simulink model "Tx_Rx_BPSK_delta_simulatie"  (Simulink 7.4)
settings: Solver=ode45  StartTime=0.0  StopTime=inf  RelTol=1e-3
undefined symbols (not defined in the file): get
libraries: dspbuff3 x16, dsparch4 x6, simulink x6, commutil2 x4, dspsrcs4 x3, commfilt2 x3, dspsnks4 x2, commchan3 x1, commsink2 x1, dspmlti4 x1, commtimrec2 x1
settings Model: Creator=wnieves  LastModifiedBy=Bscheers
settings OptimizationCC: InitFltsAndDblsToZero=on

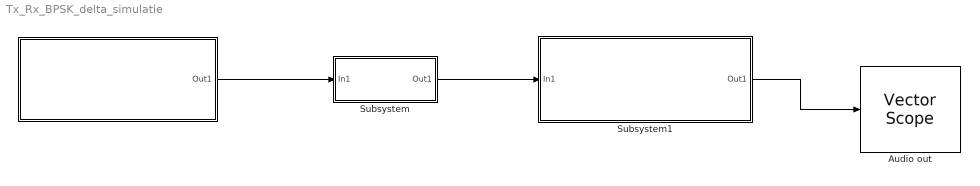
== system Tx_Rx_BPSK_delta_simulatie ==
  " " : Subsystem  Description=Transmitter
      mask Display: color('red');fprintf('Transmitter')
  Audio out : dspsnks4/Vector Scope  DialogController=dspdialog.VectorScope  DialogControllerArgs=DataTag7  ScopeProperties=on  Domain=Time  HorizSpan=1  DisplayProperties=off  AxisGrid=on  Memory=off  FrameNumber=on  AxisLegend=off  AxisZoom=off  OpenScopeAtSimStart=on  OpenScopeImmediately=off  FigPos=get(0,'defaultfigureposition')  AxisProperties=off  XUnits=Hertz  XRange=[0...Fs/2]  InheritXIncr=on  XIncr=1  XLabel=Time  XLimit=Auto  XMin=0  XMax=1  XStart=0  YUnits=dB  YLabel=Amplitude  LineProperties=off  XAxisParamsVer=6.9
      settings: YMin=-1  YMax=1
  Subsystem : Subsystem
      mask Display: fprintf('Channel')
  Subsystem1 : Subsystem
      mask Display: fprintf('Receiver')
  wires:
  " "/1(Out1) -> Subsystem/1(In1)
  Subsystem/1(Out1) -> Subsystem1/1(In1)
  Subsystem1/1(Out1) -> Audio out/1

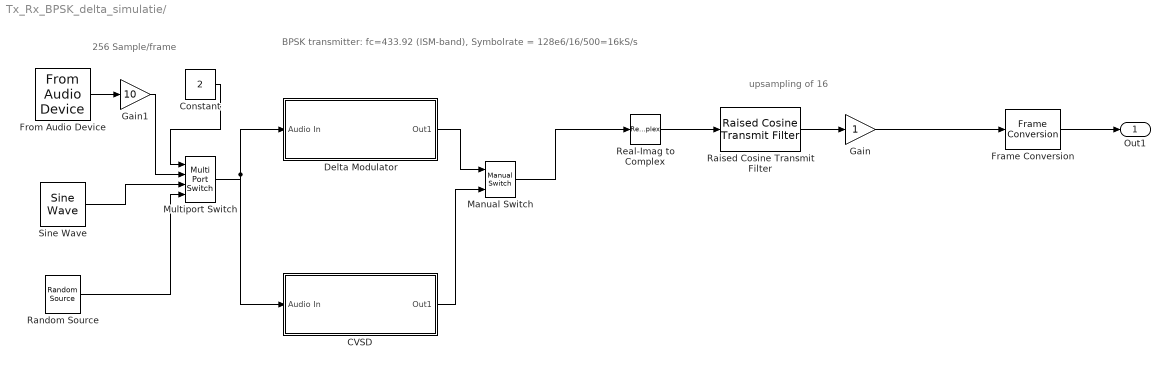
== system Tx_Rx_BPSK_delta_simulatie/  ==
  note: BPSK transmitter: fc=433.92 (ISM-band), Symbolrate = 128e6/16/500=16kS/s
  note: 256 Sample/frame
  note: upsampling of 16
  CVSD : Subsystem
  Constant : Constant  Value=2  OutDataType=fixdt(1, 16)  OutScaling=2^0
  Delta Modulator : Subsystem
  Frame Conversion : FrameConversion
  From Audio Device : dspsrcs4/From Audio Device  DialogController=dspDDGCreate  DialogControllerArgs=DataTag4  deviceName=Default  numChannels=1  sampleRate=16000  deviceDatatype=Determine from output data type  autoBufferSize=on  bufferSize=4096  queueDuration=1.0  frameSize=256  outputDatatype=single
  Gain : Gain  ParameterDataType=sfix(16)  ParameterScaling=2^0  OutDataType=sfix(16)  OutScaling=2^0
  Gain1 : Gain  Gain=10  ParameterDataType=fixdt(1, 16)  ParameterScaling=2^0  OutDataType=fixdt(1, 16)  OutScaling=2^0
  Manual Switch : simulink/Signal Routing/Manual Switch  SystemSampleTime=-1  sw=1  action=0  varsize=off
  Multiport Switch : MultiPortSwitch  OutDataType=fixdt(1, 16)  OutScaling=2^0
  Raised Cosine Transmit Filter : commfilt2/Raised Cosine Transmit Filter  DialogController=dspDDGCreate  DialogControllerArgs=DataTag5  SystemSampleTime=-1  filtType=Square root  D=8  R=0.35  sampMode=Mute  saveAsFlag=0  framing=Maintain input frame rate  N=16  checkGain=Normalized  filterGain=1  checkCoeff=off  variableName=rcTxFilt  launchFVT=off  roundingMode=Floor  overflowMode=off
  Random Source : dspsrcs4/Random Source  SrcType=Uniform  NormMethod=Ziggurat  CltLength=12  MinVal=-1  MaxVal=1  MeanVal=0  VarVal=1  RepMode=Not repeatable  rawSeed=1  IsInherit=off  SampMode=Discrete  SampTime=1/16000  SampFrame=256  DataType=Double  OutComplex=Real
  Real-Imag to Complex : RealImagToComplex  Input=Real
  Sine Wave : dspsrcs4/Sine Wave  Amplitude=1  Frequency=800  Phase=0  SampleMode=Discrete  OutComplex=Real  CompMethod=Trigonometric fcn  TableSize=Speed  SampleTime=1/16000  SamplesPerFrame=256  dataType=double  wordLen=16  udDataType=sfix(16)  fracBitsMode=Best precision  numFracBits=15  ResetState=Restart at time zero
  Out1 : Outport
  wires:
  Real-Imag to Complex/1 -> Raised Cosine Transmit Filter/1
  From Audio Device/1 -> Gain1/1
  Gain/1 -> Frame Conversion/1
  Raised Cosine Transmit Filter/1 -> Gain/1
  Delta Modulator/1(Out1) -> Manual Switch/1
  CVSD/1(Out1) -> Manual Switch/2
  Manual Switch/1 -> Real-Imag to Complex/1
  Frame Conversion/1 -> Out1/1
  Multiport Switch/1 -> Delta Modulator/1(Audio In), CVSD/1(Audio In)
  Gain1/1 -> Multiport Switch/2
  Sine Wave/1 -> Multiport Switch/3
  Random Source/1 -> Multiport Switch/4
  Constant/1 -> Multiport Switch/1

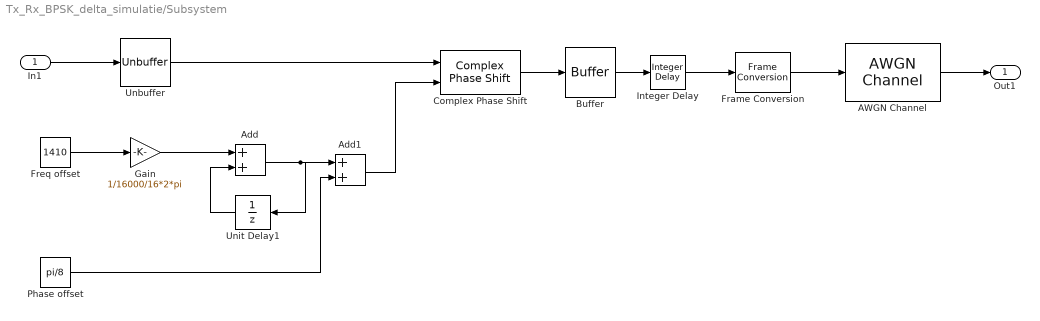
== system Tx_Rx_BPSK_delta_simulatie/Subsystem ==
  In1 : Inport  OutDataType=fixdt(1, 16)  OutScaling=2^0
  AWGN Channel : commchan3/AWGN Channel  SystemSampleTime=-1  seed=67  noiseMode="Signal to noise ratio  (SNR)"  EbNodB=20  EsNodB=10  SNRdB=20  bitsPerSym=1  Ps=1  Tsym=1  variance=1
  Add : Sum  OutDataType=fixdt(1, 16)  OutScaling=2^-10
  Add1 : Sum  OutDataType=fixdt(1, 16)  OutScaling=2^-10
  Buffer : dspbuff3/Buffer  N=4096  V=0  ic=0
  Complex Phase Shift : commutil2/Complex Phase Shift  SystemSampleTime=-1
  Frame Conversion : FrameConversion
  Freq offset : Constant  Value=1410  OutDataType=fixdt(1, 16)  OutScaling=2^0
      settings: SamplingMode=Frame based
  Gain : Gain  Gain=1/16000/16*2*pi  ParameterDataType=fixdt(1, 16)  ParameterScaling=2^0  OutDataType=fixdt(1, 16)  OutScaling=2^0
  Integer Delay : simulink/Discrete/Integer Delay  vinit=0.0  samptime=-1  NumDelays=4
  Phase offset : Constant  Value=pi/8  OutDataType=fixdt(1, 16)  OutScaling=2^0
      settings: SamplingMode=Frame based
  Unbuffer : dspbuff3/Unbuffer  ic=0
  Unit Delay1 : UnitDelay  SampleTime=-1
  Out1 : Outport  OutDataType=fixdt(1, 16)  OutScaling=2^0
  wires:
  Integer Delay/1 -> Frame Conversion/1
  Frame Conversion/1 -> AWGN Channel/1
  Complex Phase Shift/1 -> Buffer/1
  In1/1 -> Unbuffer/1
  Freq offset/1 -> Gain/1
  Gain/1 -> Add/1
  Add/1 -> Unit Delay1/1, Add1/1
  Unit Delay1/1 -> Add/2
  Phase offset/1 -> Add1/2
  Unbuffer/1 -> Complex Phase Shift/1
  Add1/1 -> Complex Phase Shift/2
  Buffer/1 -> Integer Delay/1
  AWGN Channel/1 -> Out1/1

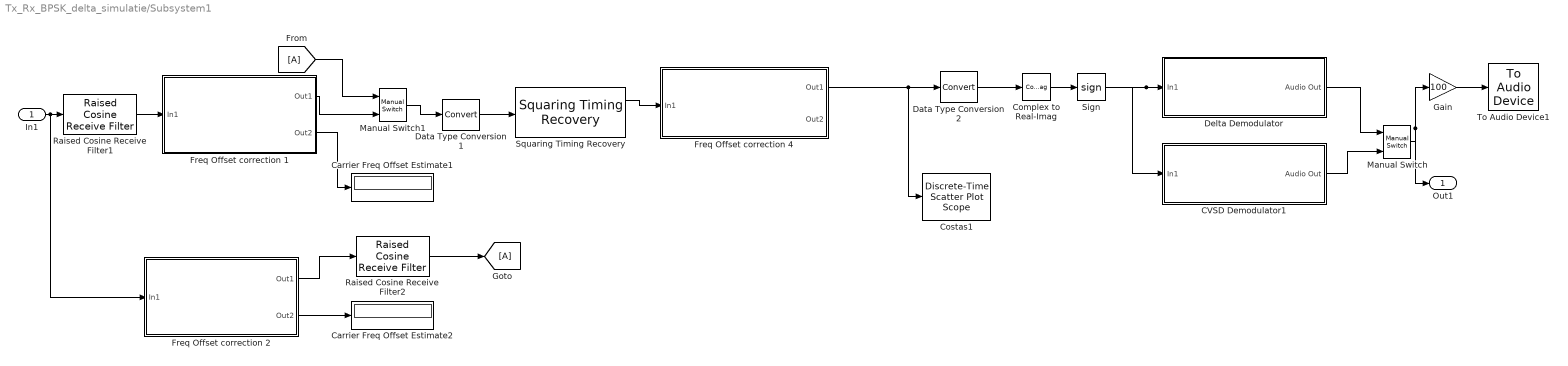
== system Tx_Rx_BPSK_delta_simulatie/Subsystem1 ==
  In1 : Inport  OutDataType=fixdt(1, 16)  OutScaling=2^0
  CVSD Demodulator1 : Subsystem
  Carrier Freq Offset Estimate1 : Display
  Carrier Freq Offset Estimate2 : Display
  Complex to Real-Imag : ComplexToRealImag  Output=Real
  Costas1 : commsink2/Discrete-Time Scatter Plot Scope  Tag=ScatterPlot  SystemSampleTime=-1  sampPerSymb=1  offsetEye=0  numTraces=40  numNewFrames=10  LineMarkers=.  LineColors=b  fading=on  render=on  AxisGrid=on  xMin=-1.60978085285153  xMax=1.62663894428818  yMin=-1.63581285423745  yMax=1.60060694290226  inphaseLabel=In-phase Amplitude  quadratureLabel=Quadrature Amplitude  openScopeAtSimStart=on  FrameNumber=off  FigPos=get(0,'defaultfigureposition');  figTitle=Scatter Plot  numLinesMax=8  block_type_=scatter
  Data Type Conversion1 : DataTypeConversion  OutDataType=fixdt(1, 16)  OutScaling=2^0
  Data Type Conversion2 : DataTypeConversion  OutDataType=fixdt(1, 16)  OutScaling=2^0
  Delta Demodulator : Subsystem
  Freq Offset correction 1 : Subsystem
      mask Display: fprintf('Delay and Multiply');
  Freq Offset correction 2 : Subsystem
      mask Display: fprintf('Coarse Freq Offset Estimater \n Delay-and-Multiply')
  Freq Offset correction 4 : Subsystem
      mask Display: fprintf('Costas Loop');
  Gain : Gain  Gain=100  ParameterDataType=fixdt(1, 16)  ParameterScaling=2^0  OutDataType=fixdt(1, 16)  OutScaling=2^0
  Manual Switch : simulink/Signal Routing/Manual Switch  SystemSampleTime=-1  sw=1  action=0  varsize=off
  Manual Switch1 : simulink/Signal Routing/Manual Switch  SystemSampleTime=-1  sw=0  action=0  varsize=off
  Raised Cosine Receive Filter1 : commfilt2/Raised Cosine Receive Filter  DialogController=dspDDGCreate  DialogControllerArgs=DataTag11  SystemSampleTime=-1  filtType=Square root  N=16  D=8  R=0.35  sampMode=Mute  saveAsFlag=0  framing=Maintain input frame rate  rateMode=None  downFactor=8  downOffset=0  checkGain=Normalized  filterGain=1  checkCoeff=off  variableName=rcRxFilt1  launchFVT=off  roundingMode=Floor  overflowMode=off
  Raised Cosine Receive Filter2 : commfilt2/Raised Cosine Receive Filter  DialogController=dspDDGCreate  DialogControllerArgs=DataTag12  SystemSampleTime=-1  filtType=Square root  N=16  D=8  R=0.35  sampMode=Mute  saveAsFlag=0  framing=Maintain input frame rate  rateMode=None  downFactor=8  downOffset=0  checkGain=Normalized  filterGain=1  checkCoeff=off  variableName=rcRxFilt2  launchFVT=off  roundingMode=Floor  overflowMode=off
  Sign : Signum
  Squaring Timing Recovery : commtimrec2/Squaring Timing Recovery  SystemSampleTime=-1  numSymb=256  sampPerSymb=16
  To Audio Device1 : dspsnks4/To Audio Device  DialogController=dspDDGCreate  DialogControllerArgs=DataTag13  deviceName=Default  inheritSampleRate=off  sampleRate=16000  deviceDatatype=Determine from input data type  autoBufferSize=on  bufferSize=4096  queueDuration=1.0
  Out1 : Outport  OutDataType=fixdt(1, 16)  OutScaling=2^0
  wires:
  Gain/1 -> To Audio Device1/1
  Delta Demodulator/1(Audio Out) -> Manual Switch/1
  Complex to Real-Imag/1 -> Sign/1
  Sign/1 -> Delta Demodulator/1(In1), CVSD Demodulator1/1(In1)
  Manual Switch/1 -> Gain/1, Out1/1
  CVSD Demodulator1/1(Audio Out) -> Manual Switch/2
  In1/1 -> Raised Cosine Receive Filter1/1, Freq Offset correction 2/1(In1)
  Freq Offset correction 1/2(Out2) -> Carrier Freq Offset Estimate1/1
  Freq Offset correction 2/2(Out2) -> Carrier Freq Offset Estimate2/1
  Raised Cosine Receive Filter1/1 -> Freq Offset correction 1/1(In1)
  Data Type Conversion1/1 -> Squaring Timing Recovery/1
  Freq Offset correction 2/1(Out1) -> Raised Cosine Receive Filter2/1
  Raised Cosine Receive Filter2/1 -> [A]
  Freq Offset correction 1/1(Out1) -> Manual Switch1/2
  Manual Switch1/1 -> Data Type Conversion1/1
  [A] -> Manual Switch1/1
  Freq Offset correction 4/1(Out1) -> Costas1/1, Data Type Conversion2/1
  Data Type Conversion2/1 -> Complex to Real-Imag/1
  Squaring Timing Recovery/1 -> Freq Offset correction 4/1(In1)

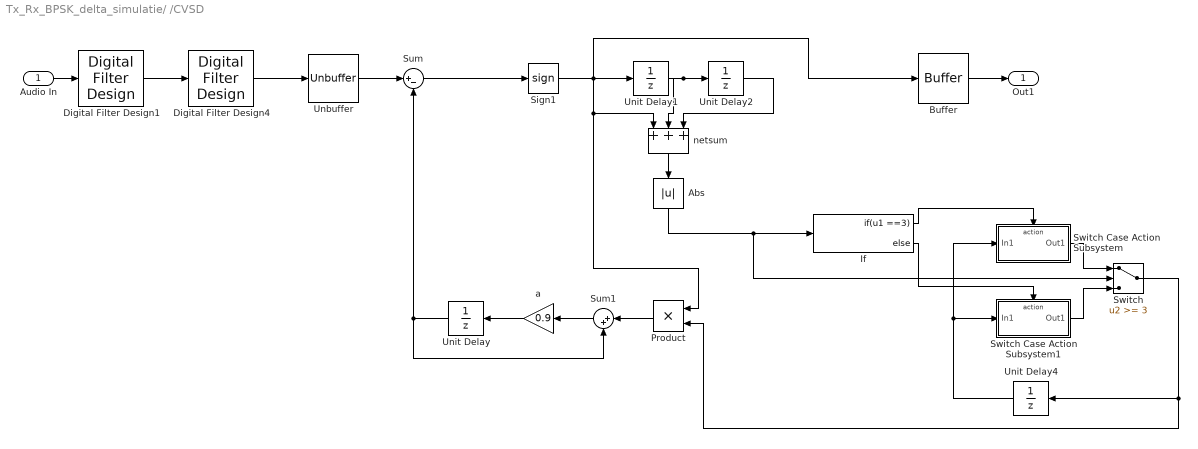
== system Tx_Rx_BPSK_delta_simulatie/ /CVSD ==
  Audio In : Inport
  Abs : Abs  OutDataType=fixdt(1, 16)  OutScaling=2^0
  Buffer : dspbuff3/Buffer  N=256  V=0  ic=0
  Digital Filter Design1 : dsparch4/Digital Filter Design  SystemSampleTime=-1  mwdsp_browser_bugfix_var=off
  Digital Filter Design4 : dsparch4/Digital Filter Design  SystemSampleTime=-1  mwdsp_browser_bugfix_var=off
  If : If  IfExpression=u1 ==3
  Product : Product  OutDataType=fixdt(1, 16)  OutScaling=2^0  RndMeth=Zero
  Sign1 : Signum
  Sum : Sum  Inputs=|+-  OutDataType=sfix(16)  OutScaling=2^0
  Sum1 : Sum  Inputs=|++  OutDataType=sfix(16)  OutScaling=2^0
  Switch : Switch  Threshold=3  OutDataType=fixdt(1, 16)  OutScaling=2^0
  Switch Case Action Subsystem : Subsystem  TreatAsAtomicUnit=on
  Switch Case Action Subsystem1 : Subsystem  TreatAsAtomicUnit=on
  Unbuffer : dspbuff3/Unbuffer  ic=0
  Unit Delay{,1..2,4} (4 alike) : UnitDelay  SampleTime=-1
  a : Gain  Gain=0.9  ParameterDataType=sfix(16)  ParameterScaling=2^0  OutDataType=sfix(16)  OutScaling=2^0
  netsum : Sum  Inputs=3  OutDataType=sfix(16)  OutScaling=2^0  SaturateOnIntegerOverflow=on  InputSameDT=on  OutDataTypeStr=Inherit: Same as first input
  Out1 : Outport
  wires:
  Sum/1 -> Sign1/1
  Sign1/1 -> Unit Delay1/1, netsum/1, Product/1, Buffer/1
  Sum1/1 -> a/1
  a/1 -> Unit Delay/1
  Unit Delay/1 -> Sum1/2, Sum/2
  Digital Filter Design1/1 -> Digital Filter Design4/1
  Digital Filter Design4/1 -> Unbuffer/1
  Unbuffer/1 -> Sum/1
  Buffer/1 -> Out1/1
  Audio In/1 -> Digital Filter Design1/1
  Unit Delay1/1 -> Unit Delay2/1, netsum/2
  Unit Delay2/1 -> netsum/3
  netsum/1 -> Abs/1
  Abs/1 -> If/1, Switch/2
  If/1 -> Switch Case Action Subsystem/Action
  Unit Delay4/1 -> Switch Case Action Subsystem1/1(In1), Switch Case Action Subsystem/1(In1)
  If/2 -> Switch Case Action Subsystem1/Action
  Switch Case Action Subsystem/1(Out1) -> Switch/1
  Switch Case Action Subsystem1/1(Out1) -> Switch/3
  Switch/1 -> Unit Delay4/1, Product/2
  Product/1 -> Sum1/1

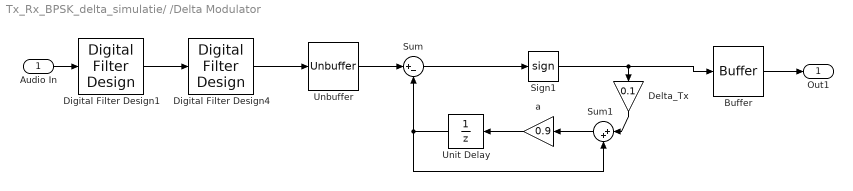
== system Tx_Rx_BPSK_delta_simulatie/ /Delta Modulator ==
  Audio In : Inport
  Buffer : dspbuff3/Buffer  N=256  V=0  ic=0
  Delta_Tx : Gain  Gain=0.1  ParameterDataType=sfix(16)  ParameterScaling=2^0  OutDataType=sfix(16)  OutScaling=2^0
  Digital Filter Design1 : dsparch4/Digital Filter Design  SystemSampleTime=-1  mwdsp_browser_bugfix_var=off
  Digital Filter Design4 : dsparch4/Digital Filter Design  SystemSampleTime=-1  mwdsp_browser_bugfix_var=off
  Sign1 : Signum
  Sum : Sum  Inputs=|+-  OutDataType=sfix(16)  OutScaling=2^0
  Sum1 : Sum  Inputs=|++  OutDataType=sfix(16)  OutScaling=2^0
  Unbuffer : dspbuff3/Unbuffer  ic=0
  Unit Delay : UnitDelay  SampleTime=-1
  a : Gain  Gain=0.9  ParameterDataType=sfix(16)  ParameterScaling=2^0  OutDataType=sfix(16)  OutScaling=2^0
  Out1 : Outport
  wires:
  Sum/1 -> Sign1/1
  Sign1/1 -> Delta_Tx/1, Buffer/1
  Delta_Tx/1 -> Sum1/1
  Sum1/1 -> a/1
  a/1 -> Unit Delay/1
  Unit Delay/1 -> Sum1/2, Sum/2
  Digital Filter Design1/1 -> Digital Filter Design4/1
  Digital Filter Design4/1 -> Unbuffer/1
  Unbuffer/1 -> Sum/1
  Buffer/1 -> Out1/1
  Audio In/1 -> Digital Filter Design1/1

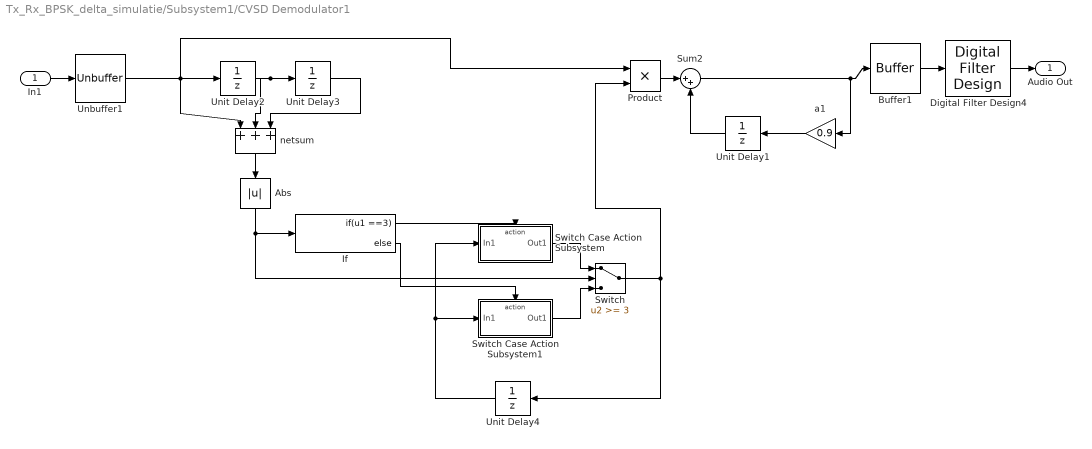
== system Tx_Rx_BPSK_delta_simulatie/Subsystem1/CVSD Demodulator1 ==
  In1 : Inport
  Abs : Abs  OutDataType=fixdt(1, 16)  OutScaling=2^0
  Buffer1 : dspbuff3/Buffer  N=256  V=0  ic=0
  Digital Filter Design4 : dsparch4/Digital Filter Design  SystemSampleTime=-1  mwdsp_browser_bugfix_var=off
  If : If  IfExpression=u1 ==3
  Product : Product  OutDataType=fixdt(1, 16)  OutScaling=2^0  RndMeth=Zero
  Sum2 : Sum  Inputs=|++  OutDataType=sfix(16)  OutScaling=2^0
  Switch : Switch  Threshold=3  OutDataType=fixdt(1, 16)  OutScaling=2^0
  Switch Case Action Subsystem : Subsystem  TreatAsAtomicUnit=on
  Switch Case Action Subsystem1 : Subsystem  TreatAsAtomicUnit=on
  Unbuffer1 : dspbuff3/Unbuffer  ic=0
  Unit Delay{1..4} (4 alike) : UnitDelay  SampleTime=-1
  a1 : Gain  Gain=0.9  ParameterDataType=sfix(16)  ParameterScaling=2^0  OutDataType=sfix(16)  OutScaling=2^0
  netsum : Sum  Inputs=3  OutDataType=sfix(16)  OutScaling=2^0  SaturateOnIntegerOverflow=on  InputSameDT=on  OutDataTypeStr=Inherit: Same as first input
  Audio Out : Outport
  wires:
  Product/1 -> Sum2/1
  a1/1 -> Unit Delay1/1
  Unit Delay1/1 -> Sum2/2
  Sum2/1 -> a1/1, Buffer1/1
  Unbuffer1/1 -> Unit Delay2/1, netsum/1, Product/1
  In1/1 -> Unbuffer1/1
  Buffer1/1 -> Digital Filter Design4/1
  Unit Delay2/1 -> Unit Delay3/1, netsum/2
  Unit Delay3/1 -> netsum/3
  netsum/1 -> Abs/1
  Abs/1 -> If/1, Switch/2
  If/1 -> Switch Case Action Subsystem/Action
  Unit Delay4/1 -> Switch Case Action Subsystem1/1(In1), Switch Case Action Subsystem/1(In1)
  If/2 -> Switch Case Action Subsystem1/Action
  Switch Case Action Subsystem/1(Out1) -> Switch/1
  Switch Case Action Subsystem1/1(Out1) -> Switch/3
  Switch/1 -> Unit Delay4/1, Product/2
  Digital Filter Design4/1 -> Audio Out/1

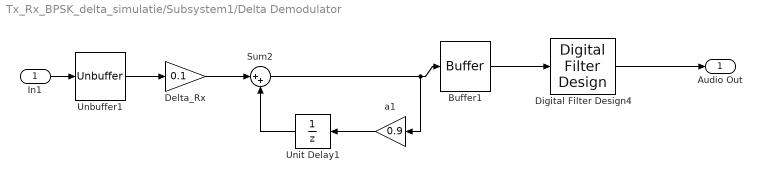
== system Tx_Rx_BPSK_delta_simulatie/Subsystem1/Delta Demodulator ==
  In1 : Inport
  Buffer1 : dspbuff3/Buffer  N=256  V=0  ic=0
  Delta_Rx : Gain  Gain=0.1  ParameterDataType=sfix(16)  ParameterScaling=2^0  OutDataType=sfix(16)  OutScaling=2^0
  Digital Filter Design4 : dsparch4/Digital Filter Design  SystemSampleTime=-1  mwdsp_browser_bugfix_var=off
  Sum2 : Sum  Inputs=|++  OutDataType=sfix(16)  OutScaling=2^0
  Unbuffer1 : dspbuff3/Unbuffer  ic=0
  Unit Delay1 : UnitDelay  SampleTime=-1
  a1 : Gain  Gain=0.9  ParameterDataType=sfix(16)  ParameterScaling=2^0  OutDataType=sfix(16)  OutScaling=2^0
  Audio Out : Outport
  wires:
  Delta_Rx/1 -> Sum2/1
  a1/1 -> Unit Delay1/1
  Unit Delay1/1 -> Sum2/2
  Sum2/1 -> a1/1, Buffer1/1
  Unbuffer1/1 -> Delta_Rx/1
  In1/1 -> Unbuffer1/1
  Buffer1/1 -> Digital Filter Design4/1
  Digital Filter Design4/1 -> Audio Out/1

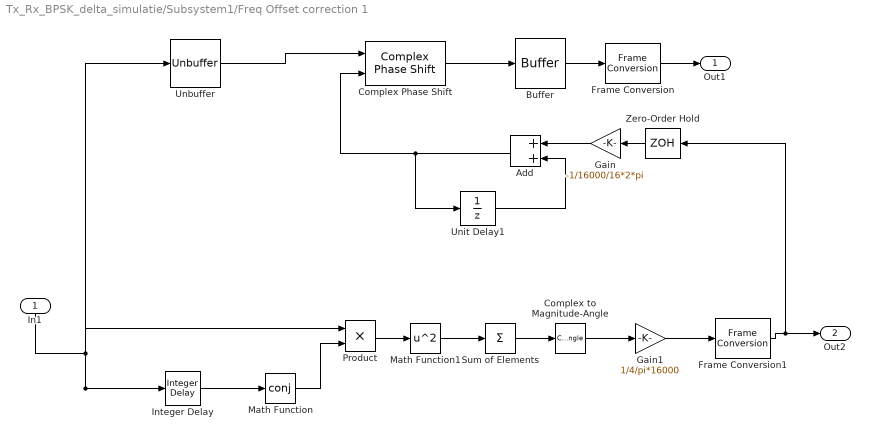
== system Tx_Rx_BPSK_delta_simulatie/Subsystem1/Freq Offset correction 1 ==
  In1 : Inport
  Add : Sum  OutDataType=fixdt(1, 16)  OutScaling=2^-10
  Buffer : dspbuff3/Buffer  N=4096  V=0  ic=0
  Complex Phase Shift : commutil2/Complex Phase Shift  SystemSampleTime=-1
  Complex to Magnitude-Angle : ComplexToMagnitudeAngle  Output=Angle
  Frame Conversion : FrameConversion
  Frame Conversion1 : FrameConversion  OutFrame=Sample-based
  Gain : Gain  Gain=-1/16000/16*2*pi  ParameterDataType=fixdt(1, 16)  ParameterScaling=2^0  OutDataType=fixdt(1, 16)  OutScaling=2^0
  Gain1 : Gain  Gain=1/4/pi*16000  ParameterDataType=fixdt(1, 16)  ParameterScaling=2^0  OutDataType=fixdt(1, 16)  OutScaling=2^0
  Integer Delay : simulink/Discrete/Integer Delay  vinit=0.0  samptime=-1  NumDelays=16
  Math Function : Math  Operator=conj  OutDataType=fixdt(1, 16)  OutScaling=2^0  SaturateOnIntegerOverflow=on
  Math Function1 : Math  Operator=square  OutDataType=fixdt(1, 16)  OutScaling=2^0  SaturateOnIntegerOverflow=on
  Product : Product  OutDataType=fixdt(1, 16)  OutScaling=2^0  RndMeth=Zero
  Sum of Elements : Sum  Inputs=+  OutDataType=fixdt(1, 16)  OutScaling=2^-10
  Unbuffer : dspbuff3/Unbuffer  ic=0
  Unit Delay1 : UnitDelay  SampleTime=-1
  Zero-Order Hold : ZeroOrderHold  SampleTime=1/16000/16
  Out1 : Outport
  Out2 : Outport  Port=2
  wires:
  Frame Conversion/1 -> Out1/1
  Frame Conversion1/1 -> Out2/1, Zero-Order Hold/1
  Gain1/1 -> Frame Conversion1/1
  In1/1 -> Integer Delay/1, Unbuffer/1, Product/1
  Complex to Magnitude-Angle/1 -> Gain1/1
  Sum of Elements/1 -> Complex to Magnitude-Angle/1
  Math Function1/1 -> Sum of Elements/1
  Product/1 -> Math Function1/1
  Math Function/1 -> Product/2
  Integer Delay/1 -> Math Function/1
  Unbuffer/1 -> Complex Phase Shift/1
  Complex Phase Shift/1 -> Buffer/1
  Buffer/1 -> Frame Conversion/1
  Gain/1 -> Add/1
  Add/1 -> Unit Delay1/1, Complex Phase Shift/2
  Unit Delay1/1 -> Add/2
  Zero-Order Hold/1 -> Gain/1

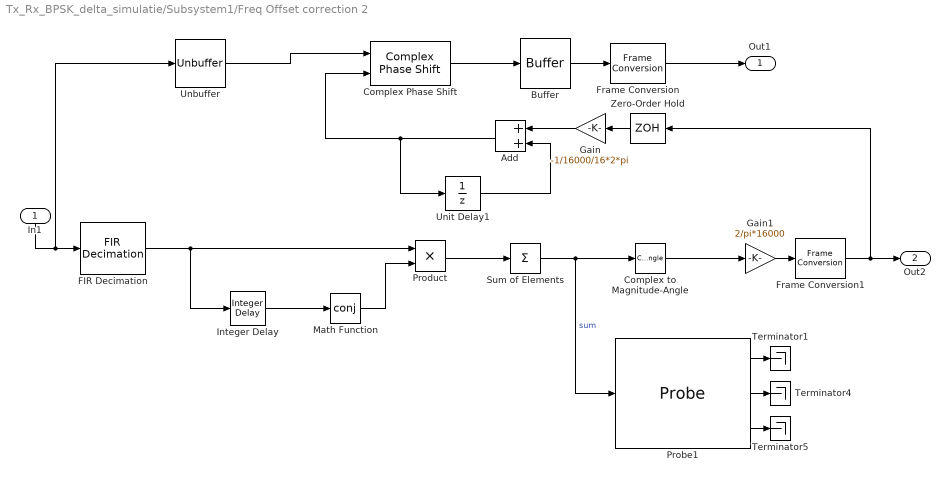
== system Tx_Rx_BPSK_delta_simulatie/Subsystem1/Freq Offset correction 2 ==
  In1 : Inport
  Add : Sum  OutDataType=fixdt(1, 16)  OutScaling=2^-10
  Buffer : dspbuff3/Buffer  N=4096  V=0  ic=0
  Complex Phase Shift : commutil2/Complex Phase Shift  SystemSampleTime=-1
  Complex to Magnitude-Angle : ComplexToMagnitudeAngle  Output=Angle
  FIR Decimation : dspmlti4/FIR Decimation  DialogController=dspdialog.FIRDecimation  DialogControllerArgs=DataTag10  h=fir1(35,0.25)  D=4  filtStruct=Direct form  framing=Maintain input frame rate  outputBufInitCond=0  roundingMode=Floor  overflowMode=off  FilterSource=Specify via dialog  FilterObject=Hm_firdecim
  Frame Conversion : FrameConversion
  Frame Conversion1 : FrameConversion  OutFrame=Sample-based
  Gain : Gain  Gain=-1/16000/16*2*pi  ParameterDataType=fixdt(1, 16)  ParameterScaling=2^0  OutDataType=fixdt(1, 16)  OutScaling=2^0
  Gain1 : Gain  Gain=2/pi*16000  ParameterDataType=fixdt(1, 16)  ParameterScaling=2^0  OutDataType=fixdt(1, 16)  OutScaling=2^0
  Integer Delay : simulink/Discrete/Integer Delay  vinit=0.0  samptime=-1  NumDelays=1
  Math Function : Math  Operator=conj  OutDataType=fixdt(1, 16)  OutScaling=2^0  SaturateOnIntegerOverflow=on
  Probe1 : Probe  ProbeComplexSignal=off  ProbeFramedSignal=on
  Product : Product  OutDataType=fixdt(1, 16)  OutScaling=2^0  RndMeth=Zero
  Sum of Elements : Sum  Inputs=+  OutDataType=fixdt(1, 16)  OutScaling=2^-10
  Terminator1 : Terminator
  Terminator4 : Terminator
  Terminator5 : Terminator
  Unbuffer : dspbuff3/Unbuffer  ic=0
  Unit Delay1 : UnitDelay  SampleTime=-1
  Zero-Order Hold : ZeroOrderHold  SampleTime=1/16000/16
  Out1 : Outport
  Out2 : Outport  Port=2
  wires:
  Frame Conversion1/1 -> Out2/1, Zero-Order Hold/1
  Probe1/3 -> Terminator5/1
  Probe1/2 -> Terminator4/1
  Probe1/1 -> Terminator1/1
  FIR Decimation/1 -> Integer Delay/1, Product/1
  Gain1/1 -> Frame Conversion1/1
  In1/1 -> FIR Decimation/1, Unbuffer/1
  Complex to Magnitude-Angle/1 -> Gain1/1
  Sum of Elements/1 -> Probe1/1, Complex to Magnitude-Angle/1  "sum"
  Product/1 -> Sum of Elements/1
  Math Function/1 -> Product/2
  Integer Delay/1 -> Math Function/1
  Unbuffer/1 -> Complex Phase Shift/1
  Complex Phase Shift/1 -> Buffer/1
  Buffer/1 -> Frame Conversion/1
  Gain/1 -> Add/1
  Add/1 -> Unit Delay1/1, Complex Phase Shift/2
  Unit Delay1/1 -> Add/2
  Zero-Order Hold/1 -> Gain/1
  Frame Conversion/1 -> Out1/1

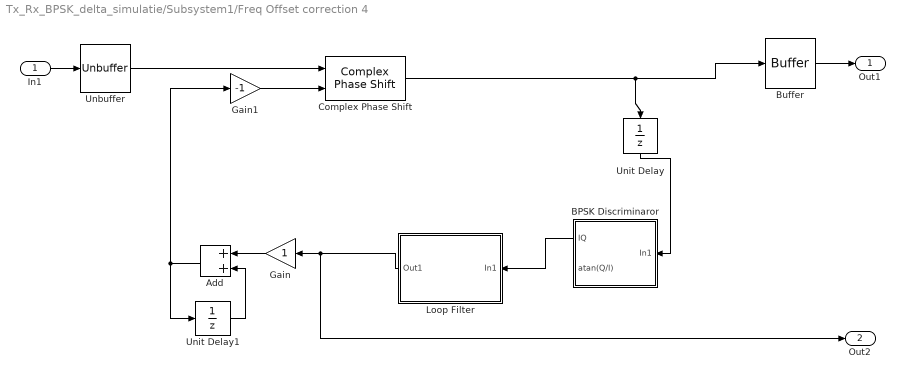
== system Tx_Rx_BPSK_delta_simulatie/Subsystem1/Freq Offset correction 4 ==
  In1 : Inport
  Add : Sum  OutDataType=fixdt(1, 16)  OutScaling=2^-10
  BPSK Discriminaror : Subsystem
  Buffer : dspbuff3/Buffer  N=256  V=0  ic=0
  Complex Phase Shift : commutil2/Complex Phase Shift  SystemSampleTime=-1
  Gain : Gain  ParameterDataType=fixdt(1, 16)  ParameterScaling=2^0  OutDataType=fixdt(1, 16)  OutScaling=2^0
  Gain1 : Gain  Gain=-1  ParameterDataType=fixdt(1, 16)  ParameterScaling=2^0  OutDataType=fixdt(1, 16)  OutScaling=2^0
  Loop Filter : Subsystem
  Unbuffer : dspbuff3/Unbuffer  ic=0
  Unit Delay : UnitDelay  SampleTime=-1
  Unit Delay1 : UnitDelay  SampleTime=-1
  Out1 : Outport
  Out2 : Outport  Port=2
  wires:
  Loop Filter/1(Out1) -> Gain/1, Out2/1
  Unit Delay/1 -> BPSK Discriminaror/1(In1)
  Complex Phase Shift/1 -> Unit Delay/1, Buffer/1
  Unbuffer/1 -> Complex Phase Shift/1
  In1/1 -> Unbuffer/1
  Buffer/1 -> Out1/1
  Add/1 -> Unit Delay1/1, Gain1/1
  Unit Delay1/1 -> Add/2
  Gain/1 -> Add/1
  Gain1/1 -> Complex Phase Shift/2
  BPSK Discriminaror/1(IQ) -> Loop Filter/1(In1)

== system Tx_Rx_BPSK_delta_simulatie/ /CVSD/Switch Case Action Subsystem ==
  In1 : Inport  OutDataType=fixdt(1, 16)  OutScaling=2^0
  Action Port : ActionPort  ActionType=then
  Constant : Constant  Value=0.5  OutDataType=fixdt(1, 16)  OutScaling=2^0
  Gain : Gain  Gain=0.7  ParameterDataType=fixdt(1, 16)  ParameterScaling=2^0  OutDataType=fixdt(1, 16)  OutScaling=2^0
  Subtract : Sum  OutDataType=fixdt(1, 16)  OutScaling=2^-10
  Out1 : Outport  OutDataType=fixdt(1, 16)  OutScaling=2^0
  wires:
  In1/1 -> Gain/1
  Gain/1 -> Subtract/1
  Constant/1 -> Subtract/2
  Subtract/1 -> Out1/1

== system Tx_Rx_BPSK_delta_simulatie/ /CVSD/Switch Case Action Subsystem1 ==
  In1 : Inport  OutDataType=fixdt(1, 16)  OutScaling=2^0
  Action Port : ActionPort  ActionType=else
  Constant : Constant  Value=0.005  OutDataType=fixdt(1, 16)  OutScaling=2^0
  Gain : Gain  Gain=0.7  ParameterDataType=fixdt(1, 16)  ParameterScaling=2^0  OutDataType=fixdt(1, 16)  OutScaling=2^0
  Subtract : Sum  OutDataType=fixdt(1, 16)  OutScaling=2^-10
  Out1 : Outport  OutDataType=fixdt(1, 16)  OutScaling=2^0
  wires:
  In1/1 -> Gain/1
  Gain/1 -> Subtract/1
  Constant/1 -> Subtract/2
  Subtract/1 -> Out1/1

== system Tx_Rx_BPSK_delta_simulatie/Subsystem1/CVSD Demodulator1/Switch Case Action Subsystem ==
  In1 : Inport  OutDataType=fixdt(1, 16)  OutScaling=2^0
  Action Port : ActionPort  ActionType=then
  Constant : Constant  Value=0.5  OutDataType=fixdt(1, 16)  OutScaling=2^0
  Gain : Gain  Gain=0.7  ParameterDataType=fixdt(1, 16)  ParameterScaling=2^0  OutDataType=fixdt(1, 16)  OutScaling=2^0
  Subtract : Sum  OutDataType=fixdt(1, 16)  OutScaling=2^-10
  Out1 : Outport  OutDataType=fixdt(1, 16)  OutScaling=2^0
  wires:
  In1/1 -> Gain/1
  Gain/1 -> Subtract/1
  Constant/1 -> Subtract/2
  Subtract/1 -> Out1/1

== system Tx_Rx_BPSK_delta_simulatie/Subsystem1/CVSD Demodulator1/Switch Case Action Subsystem1 ==
  In1 : Inport  OutDataType=fixdt(1, 16)  OutScaling=2^0
  Action Port : ActionPort  ActionType=else
  Constant : Constant  Value=0.005  OutDataType=fixdt(1, 16)  OutScaling=2^0
  Gain : Gain  Gain=0.7  ParameterDataType=fixdt(1, 16)  ParameterScaling=2^0  OutDataType=fixdt(1, 16)  OutScaling=2^0
  Subtract : Sum  OutDataType=fixdt(1, 16)  OutScaling=2^-10
  Out1 : Outport  OutDataType=fixdt(1, 16)  OutScaling=2^0
  wires:
  In1/1 -> Gain/1
  Gain/1 -> Subtract/1
  Constant/1 -> Subtract/2
  Subtract/1 -> Out1/1

== system Tx_Rx_BPSK_delta_simulatie/Subsystem1/Freq Offset correction 4/BPSK Discriminaror ==
  In1 : Inport
  Complex to Real-Imag : ComplexToRealImag
  Product : Product  OutDataType=fixdt(1, 16)  OutScaling=2^0  RndMeth=Zero
  Sign : Signum
  Trigonometric Function : Trigonometry  Operator=atan2
  IQ : Outport
  atan(Q/I) : Outport  Port=2
  wires:
  Trigonometric Function/1 -> atan(Q/I)/1
  Complex to Real-Imag/2 -> Trigonometric Function/2, Product/1
  Complex to Real-Imag/1 -> Trigonometric Function/1, Sign/1
  In1/1 -> Complex to Real-Imag/1
  Product/1 -> IQ/1
  Sign/1 -> Product/2

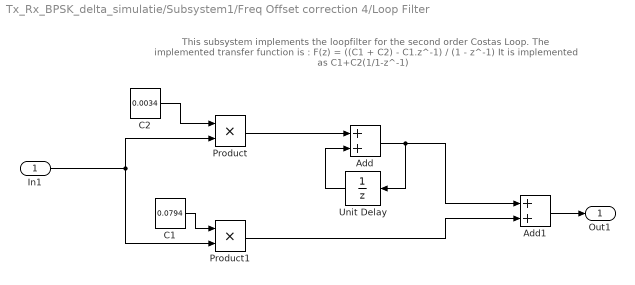
== system Tx_Rx_BPSK_delta_simulatie/Subsystem1/Freq Offset correction 4/Loop Filter ==
  note: This subsystem implements the loopfilter for the second order Costas Loop. The implemented
      | transfer function is : F(z) = ((C1 + C2) - C1.z^-1) / (1 - z^-1)
      |
      | It is implemented as C1+C2(1/1-z^-1)
  In1 : Inport  OutDataType=fixdt(1, 16)  OutScaling=2^0
  Add : Sum  OutDataType=fixdt(1, 16)  OutScaling=2^-10
  Add1 : Sum  OutDataType=fixdt(1, 16)  OutScaling=2^-10
  C1 : Constant  Value=0.0794  OutDataTypeMode=single  OutDataType=fixdt(1, 16)  OutScaling=2^0  OutDataTypeStr=single
  C2 : Constant  Value=0.0034  OutDataTypeMode=single  OutDataType=fixdt(1, 16)  OutScaling=2^0  OutDataTypeStr=single
  Product : Product  OutDataType=fixdt(1, 16)  OutScaling=2^0  RndMeth=Zero
  Product1 : Product  OutDataType=fixdt(1, 16)  OutScaling=2^0  RndMeth=Zero
  Unit Delay : UnitDelay  X0=0.1  SampleTime=-1
  Out1 : Outport  OutDataType=fixdt(1, 16)  OutScaling=2^0
  wires:
  C1/1 -> Product1/1
  Add1/1 -> Out1/1
  Unit Delay/1 -> Add/2
  Add/1 -> Unit Delay/1, Add1/1
  Product1/1 -> Add1/2
  Product/1 -> Add/1
  In1/1 -> Product1/2, Product/2
  C2/1 -> Product/1
